simulink model "propeller_arm_control"  (R2021b)
settings: Solver=VariableStepAuto  StartTime=0.0  StopTime=10.0  RelTol=1e-3
values from neighbouring files (symbols this model uses):
  N = 20    [RlocusPIDControlProject.m]
  Ts = 0.01    [RlocusPIDControlProject.m]
libraries: simulink x1
settings Model: Creator=Yusuf  LastModifiedBy=Yusuf

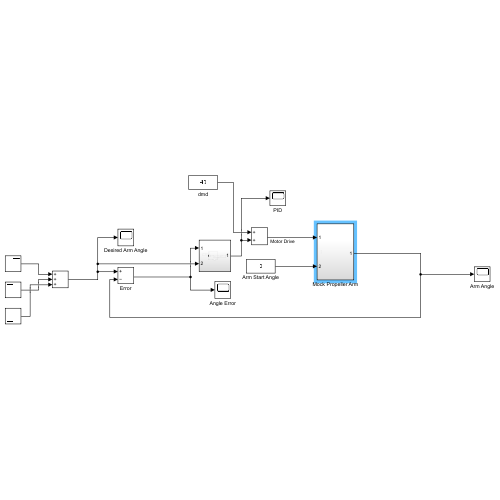
[thumbnail: Simulink's stored preview of the top-level diagram]
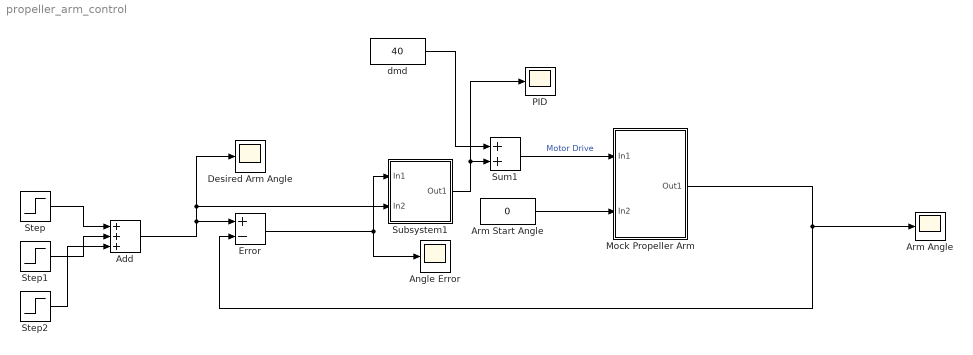
== system propeller_arm_control ==
  Add : Sum  Inputs=+++
  Angle Error : Scope
  Arm Angle : Scope
  Arm Start Angle : Constant  Value=0
  Desired Arm Angle : Scope
  Error : Sum  Inputs=+-
  Mock Propeller Arm : Subsystem
  PID : Scope
  Step : Step  After=45  SampleTime=Ts
  Step1 : Step  Time=301  After=-45  SampleTime=Ts
  Step2 : Step  Time=601  After=89.92  SampleTime=Ts
  Subsystem1 : Subsystem
  Sum1 : Sum
  dmd : Constant  Value=40
  wires:
  Sum1/1 -> Mock Propeller Arm/1(In1)  "Motor Drive"
  Subsystem1/1(Out1) -> PID/1, Sum1/2
  Step2/1 -> Add/3
  Mock Propeller Arm/1(Out1) -> Error/2, Arm Angle/1
  dmd/1 -> Sum1/1
  Step/1 -> Add/1
  Error/1 -> Subsystem1/1(In1), Angle Error/1
  Arm Start Angle/1 -> Mock Propeller Arm/2(In2)
  Add/1 -> Error/1, Subsystem1/2(In2), Desired Arm Angle/1
  Step1/1 -> Add/2

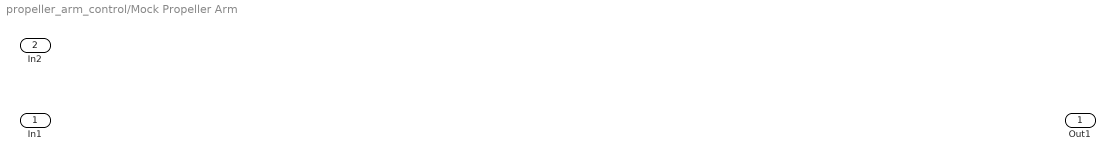
== system propeller_arm_control/Mock Propeller Arm ==
  In1 : Inport
  In2 : Inport  Port=2
  Out1 : Outport

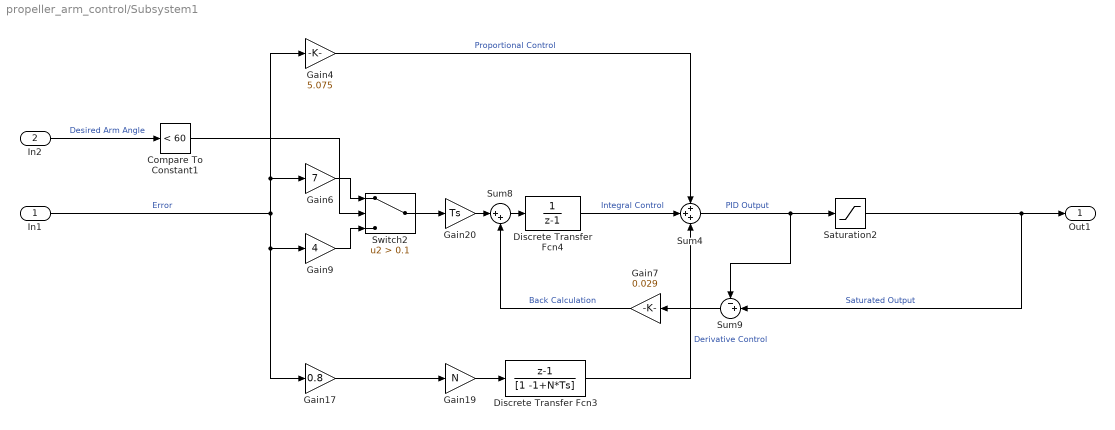
== system propeller_arm_control/Subsystem1 ==
  In1 : Inport
  In2 : Inport  Port=2
  Compare To Constant1 : simulink/Logic and Bit Operations/Compare To Constant  relop=<  const=60  OutDataTypeStr=boolean
  Discrete Transfer Fcn3 : DiscreteTransferFcn  Numerator=[1 -1]  Denominator=[1 -1+N*Ts]
  Discrete Transfer Fcn4 : DiscreteTransferFcn  Numerator=[0 1]  Denominator=[1 -1]
  Gain17 : Gain  Gain=0.8
  Gain19 : Gain  Gain=N
  Gain20 : Gain  Gain=Ts
  Gain4 : Gain  Gain=5.075
  Gain6 : Gain  Gain=7
  Gain7 : Gain  Gain=0.029
  Gain9 : Gain  Gain=4
  Saturation2 : Saturate  UpperLimit=20  LowerLimit=-75  LinearizeAsGain=off
  Sum4 : Sum  Inputs=+++
  Sum8 : Sum  Inputs=|++
  Sum9 : Sum  Inputs=-+|
  Switch2 : Switch  Criteria=u2 > Threshold  Threshold=0.1
  Out1 : Outport
  wires:
  Sum8/1 -> Discrete Transfer Fcn4/1
  Sum4/1 -> Saturation2/1, Sum9/1  "PID Output"
  Gain20/1 -> Sum8/1
  Gain19/1 -> Discrete Transfer Fcn3/1
  Switch2/1 -> Gain20/1
  Gain4/1 -> Sum4/1  "Proportional Control"
  Gain6/1 -> Switch2/1
  Compare To Constant1/1 -> Switch2/2
  Discrete Transfer Fcn4/1 -> Sum4/2  "Integral Control"
  In2/1 -> Compare To Constant1/1  "Desired Arm Angle"
  Sum9/1 -> Gain7/1
  Gain7/1 -> Sum8/2  "Back Calculation"
  In1/1 -> Gain6/1, Gain4/1, Gain9/1, Gain17/1  "Error"
  Gain9/1 -> Switch2/3
  Discrete Transfer Fcn3/1 -> Sum4/3  "Derivative Control"
  Saturation2/1 -> Sum9/2, Out1/1  "Saturated Output"
  Gain17/1 -> Gain19/1
